simulink model "lab3Synth"  (Simulink 3.00)
settings: Solver=ode45  SolverMode=SingleTasking  StartTime=0.0  StopTime=9999  MaxStep=0.005  RelTol=1e-3  AbsTol=1e-6
settings Model: RTWTemplateMakefile=grt_unix.tmf  Creator=vise  LastModifiedBy=vise

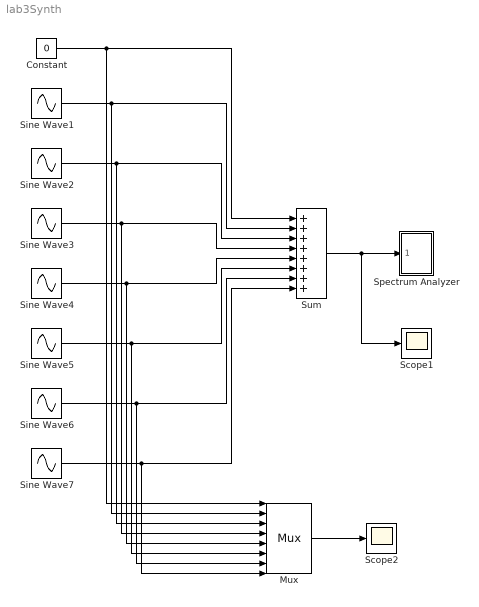
== system lab3Synth ==
  Constant : Constant  Value=0
  Mux : Mux  Inputs=8
      settings: DisplayOption=none
  Scope1 : Scope
      settings: TickLabels=on  TimeRange=2  YMin=-1.5  YMax=1.5  SaveToWorkspace=off  SaveName=ScopeData  DataFormat=Matrix
  Scope2 : Scope
      settings: TickLabels=on  TimeRange=2  YMin=-1.5  YMax=1.5  SaveToWorkspace=off  SaveName=ScopeData  DataFormat=Matrix
  Sine Wave1 : Sin  Amplitude=4/pi  Frequency=2*pi  Phase=0  SampleTime=0
  Sine Wave2 : Sin  Amplitude=4/(3*pi)  Frequency=3*2*pi  Phase=0  SampleTime=0
  Sine Wave3 : Sin  Amplitude=4/(5*pi)  Frequency=5*2*pi  Phase=0  SampleTime=0
  Sine Wave4 : Sin  Amplitude=4/(7*pi)  Frequency=7*2*pi  Phase=0  SampleTime=0
  Sine Wave5 : Sin  Amplitude=4/(9*pi)  Frequency=9*2*pi  Phase=0  SampleTime=0
  Sine Wave6 : Sin  Amplitude=4/(11*pi)  Frequency=11*2*pi  Phase=0  SampleTime=0
  Sine Wave7 : Sin  Amplitude=4/(13*pi)  Frequency=13*2*pi  Phase=0  SampleTime=0
  Spectrum Analyzer : Subsystem  mask(Spectrum analyzer.){@1=1024, @2=0.01, @3=10}
      mask prompts: @1 "Number of sample points:"; @2 "Sampling period (sec):"; @3 "Plotting Period (sec):"
      mask init:
      | N=@1; T_s=@2;plot_period=@3;
      mask Help: EE438 Lab utility; See Prof. Bouman.
      mask Display: plot(0,0,100,100,[14,91,91,14,14],[86,86,40,40,86],[85,82,80,79,75,67,63,60,57,53,41,36,33,27,24],[49,50,53,50,49,51,54,66,54,50,50,52,81,51,49])
  Sum : Sum  Inputs=++++++++  SaturateOnIntegerOverflow=on
  wires:
  Sum/1 -> Scope1/1, Spectrum Analyzer/1(input signal)
  Mux/1 -> Scope2/1
  Sine Wave7/1 -> Mux/8, Sum/8
  Sine Wave6/1 -> Mux/7, Sum/7
  Sine Wave5/1 -> Mux/6, Sum/6
  Sine Wave4/1 -> Mux/5, Sum/5
  Sine Wave3/1 -> Mux/4, Sum/4
  Sine Wave2/1 -> Mux/3, Sum/3
  Sine Wave1/1 -> Mux/2, Sum/2
  Constant/1 -> Mux/1, Sum/1

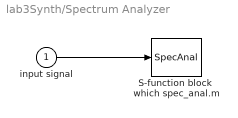
== system lab3Synth/Spectrum Analyzer ==
  input signal : Inport  Port=1  PortWidth=-1  SampleTime=-1  DataType=auto
      settings: SignalType=auto
  S-function block  which spec_anal.m : S-Function  FunctionName=SpecAnal  Parameters=N,T_s,plot_period  PortCounts=[]  SFunctionModules=''
  wires:
  input signal/1 -> S-function block  which spec_anal.m/1
